simulink model "evaporator_test"  (R2017b)
settings: Solver=VariableStepAuto  StartTime=0.0  StopTime=15000  RelTol=1e-3
settings Model: Creator=Bailey Brookes  LastModifiedBy=Bailey Brookes

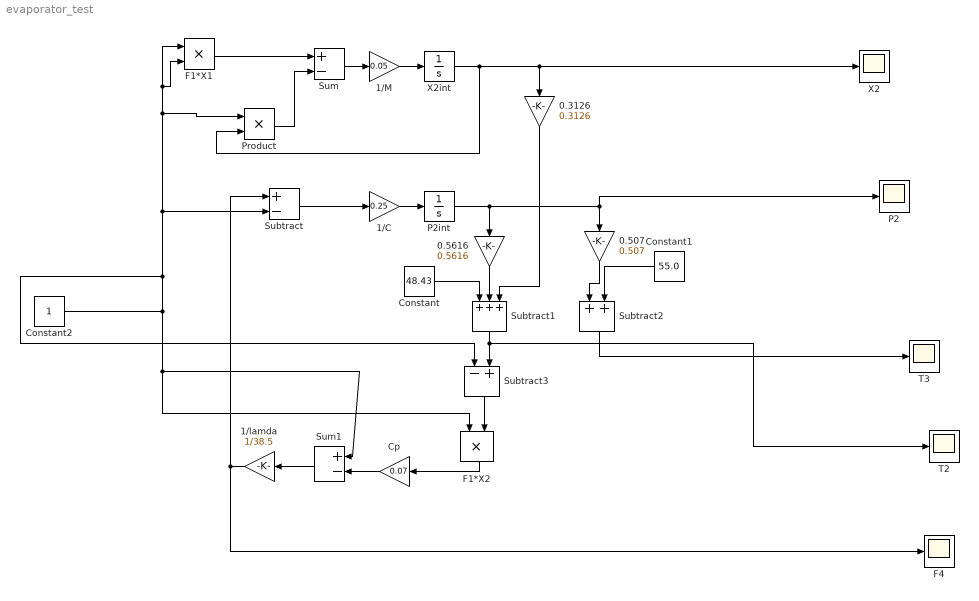
== system evaporator_test ==
  0.3126 : Gain  Gain=0.3126
  0.507 : Gain  Gain=0.507
  0.5616 : Gain  Gain=0.5616
  1/C : Gain  Gain=0.25
  1/M : Gain  Gain=0.05
  1/lamda : Gain  Gain=1/38.5
  Constant : Constant  Value=48.43
  Constant1 : Constant  Value=55.0
  Constant2 : Constant
  Cp : Gain  Gain=0.07
  F1*X1 : Product
  F1*X2 : Product
  F4 : Scope
  P2 : Scope
  P2int : Integrator
  Product : Product
  Subtract : Sum  Inputs=+-
  Subtract1 : Sum  Inputs=+++
  Subtract2 : Sum
  Subtract3 : Sum  Inputs=-+
  Sum : Sum  Inputs=+-
  Sum1 : Sum  Inputs=+-
  T2 : Scope
  T3 : Scope
  X2 : Scope
  X2int : Integrator
  wires:
  Cp/1 -> Sum1/2
  Sum1/1 -> 1/lamda/1
  Subtract1/1 -> T2/1, Subtract3/2
  0.3126/1 -> Subtract1/3
  Product/1 -> Sum/2
  X2int/1 -> X2/1, 0.3126/1, Product/2
  Constant1/1 -> Subtract2/2
  Subtract2/1 -> T3/1
  F1*X2/1 -> Cp/1
  1/M/1 -> X2int/1
  Subtract3/1 -> F1*X2/2
  Subtract/1 -> 1/C/1
  Constant/1 -> Subtract1/1
  P2int/1 -> 0.5616/1, P2/1, 0.507/1
  0.5616/1 -> Subtract1/2
  F1*X1/1 -> Sum/1
  0.507/1 -> Subtract2/1
  1/lamda/1 -> F4/1, Subtract/1
  1/C/1 -> P2int/1
  Constant2/1 -> Subtract3/1, Subtract/2, Product/1, F1*X1/2, F1*X1/1, Sum1/1, F1*X2/1
  Sum/1 -> 1/M/1
